simulink model "HCS_function_blocks"  (R2023a)
settings: Solver=ode23t  StartTime=0.0  StopTime=10  RelTol=1e-3
undefined symbols (not defined in the file): Down, Up
libraries: eePwmGenerator x1, spspowerguiLib x1
settings Model: NumberOfSteps=1000  PacingRate=89  Creator=Matt Smith  LastModifiedBy=matty

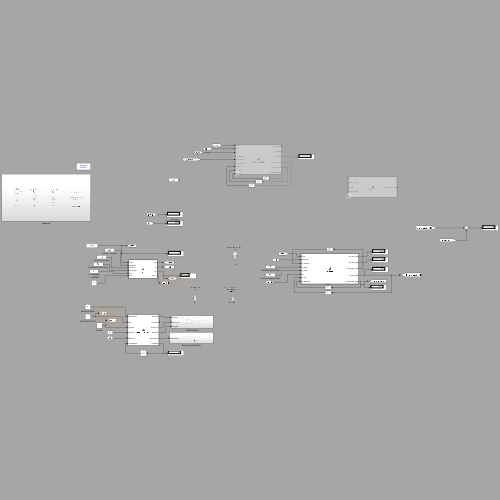
[thumbnail: Simulink's stored preview of the top-level diagram]
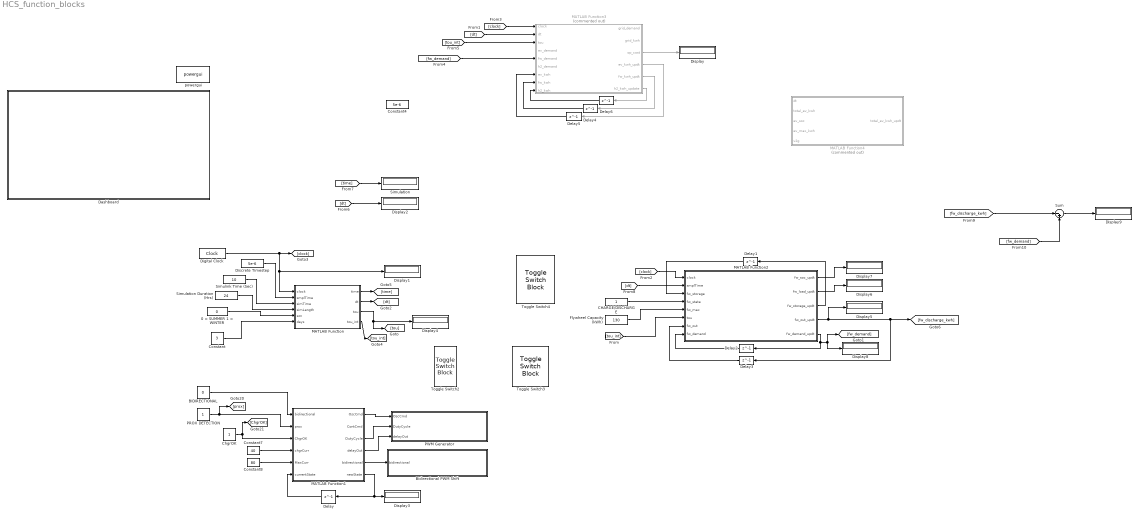
== system HCS_function_blocks ==
  0 = SUMMER 1 = WINTER : Constant  Value=0
  BIDIRECTIONAL : Constant  Value=0
  Bidirectional PWM Shift : Subsystem
  CHARGE/DISCHARGE : Constant
  ChgrOK : Constant
  Constant : Constant  Value=3
  Constant4 : Constant  Value=5e-6
  Constant7 : Constant  Value=40
  Constant8 : Constant  Value=80
  Dashboard : Subsystem
  Delay : Delay  DelayLength=1  InitialCondition=0
  Delay{1..6} (6 alike) : Delay  DelayLength=1  SampleTime=5e-6
  Digital Clock : DigitalClock  SampleTime=5e-6
  Discrete Timestep : Constant  Value=5e-6
  Display{,1..9} (10 alike) : Display
  Flywheel Capacity (kWh) : Constant  Value=130
  MATLAB Function : MATLAB Function  TreatAsAtomicUnit=on
  MATLAB Function1 : MATLAB Function  TreatAsAtomicUnit=on
  MATLAB Function2 : MATLAB Function  TreatAsAtomicUnit=on
  MATLAB Function3 : MATLAB Function  Commented=on  TreatAsAtomicUnit=on
  MATLAB Function4 : MATLAB Function  Commented=on  TreatAsAtomicUnit=on
  PROX DETECTION : Constant
  PWM Generator : Subsystem
  Simulation : Display
  Simulation Duration (Hrs) : Constant  Value=24
  Simulink Time (Sec) : Constant  Value=10
  Sum : Sum  Inputs=|-+
  Toggle Switch2 : ToggleSwitchBlock
      settings: Values={{'Off', 'On'}, [0 1]}
  Toggle Switch3 : ToggleSwitchBlock
      settings: Values={{'SUMMER', 'WINTER'}, [0 1]}
  Toggle Switch4 : ToggleSwitchBlock
      settings: Values={{'Off', 'On'}, [-1 1]}
  powergui : spspowerguiLib/powergui  Priority=1  SimulationMode=Discrete  SampleTime=5e-6  frequency=60  Iterations=50  frequencyindice=0  Pbase=100e6  ErrMax=1e-4  UnitsV=kV  UnitsW=MW  buscounter=0  FunctionMessages=off  echomessages=off  EnableUseOfTLC=off  CurrentSourceSwitches=off  DisableSnubberDevices=off  DisableRonSwitches=off  DisableVfSwitches=off  DisplayEquations=off  AutomaticDiscreteSolvers=off  SolverType=Tustin/Backward Euler (TBE)  Interpol=off  ExternalGateDelay=off  methode=off  Ts=100  x0status=blocks  SPID=on  SwTol=0  HookPort=off  NonlinearTolerance=1e-4  nMaxIteration=100  ContinueOnMaxIteration=off  RestoreLinks=warning  ResistiveCurrentMeasurement=off  Frange=[0:2:500]  Ylog=off  Xlog=on  ShowGrid=off  save=off  variable=ZData  structure=0  ZoomFFT=off  StartTime=0.0  cycles=1  DisplayStyle=1  fundamental=60  FreqAxis=off  MaxFrequency=1000  frequencyindicesteady=1  RmsSteady=1  display=off
  wires:
  Constant8/1 -> MATLAB Function1/5(MaxCurr)
  PROX DETECTION/1 -> MATLAB Function1/2(prox), [prox]
  Constant7/1 -> MATLAB Function1/4(chgrCurr)
  BIDIRECTIONAL/1 -> MATLAB Function1/1("bidirectional ")
  Delay/1 -> MATLAB Function1/6(currentState)
  ChgrOK/1 -> [ChgrOK], MATLAB Function1/3(ChgrOK)
  MATLAB Function1/6(newState) -> Delay/1, Display3/1
  MATLAB Function1/5(bidirectional) -> Bidirectional PWM Shift/1(bidirectional)
  MATLAB Function1/1(OscCmd) -> PWM Generator/1(OscCmd)
  MATLAB Function1/4(delayOut) -> PWM Generator/3(delayOut)
  MATLAB Function1/3(DutyCycle) -> PWM Generator/2(DutyCycle)
  Digital Clock/1 -> [clock], MATLAB Function/1(clock), Display1/1
  Discrete Timestep/1 -> MATLAB Function/2(smplTime)
  MATLAB Function/3(tou) -> [tou], Display4/1
  Simulink Time (Sec)/1 -> MATLAB Function/3(simTime)
  Simulation Duration (Hrs)/1 -> MATLAB Function/4(simLength)
  0 = SUMMER 1 = WINTER/1 -> MATLAB Function/5(szn)
  [tou_int] -> MATLAB Function2/6(tou)
  MATLAB Function2/3(fw_storage_updt) -> Delay1/1
  Delay1/1 -> MATLAB Function2/3(fw_storage)
  Flywheel Capacity (kWh)/1 -> MATLAB Function2/5(fw_max)
  MATLAB Function2/4(fw_out_updt) -> [fw_discharge_kwh], Delay3/1, Display5/1
  MATLAB Function2/2(fw_load_updt) -> Display6/1
  MATLAB Function2/1(fw_soc_updt) -> Display7/1
  MATLAB Function2/5(fw_demand_updt) -> Delay2/1, [fw_demand], Display8/1
  MATLAB Function/2(dt) -> [dt]
  [clock] -> MATLAB Function2/1(clock)
  Delay2/1 -> MATLAB Function2/8(fw_demand)
  Constant/1 -> MATLAB Function/6(days)
  CHARGE/DISCHARGE/1 -> MATLAB Function2/4(fw_state)
  MATLAB Function/4(tou_int) -> [tou_int]
  [dt] -> MATLAB Function3/2(dt)
  [tou_int] -> MATLAB Function3/3(tou)
  [fw_demand] -> MATLAB Function3/5(fw_demand)
  MATLAB Function3/3(op_cost) -> Display/1
  [clock] -> MATLAB Function3/1(clock)
  [dt] -> Display2/1
  MATLAB Function/1(time) -> [time]
  [time] -> Simulation/1
  [dt] -> MATLAB Function2/2(smplTime)
  Delay3/1 -> MATLAB Function2/7(fw_out)
  [fw_discharge_kwh] -> Sum/1
  [fw_demand] -> Sum/2
  Sum/1 -> Display9/1
  MATLAB Function3/4(ev_kwh_updt) -> Delay5/1
  Delay5/1 -> MATLAB Function3/7(ev_kwh)
  MATLAB Function3/5(fw_kwh_updt) -> Delay4/1
  Delay4/1 -> MATLAB Function3/8(fw_kwh)
  MATLAB Function3/6(h2_kwh_update) -> Delay6/1
  Delay6/1 -> MATLAB Function3/9(h2_kwh)

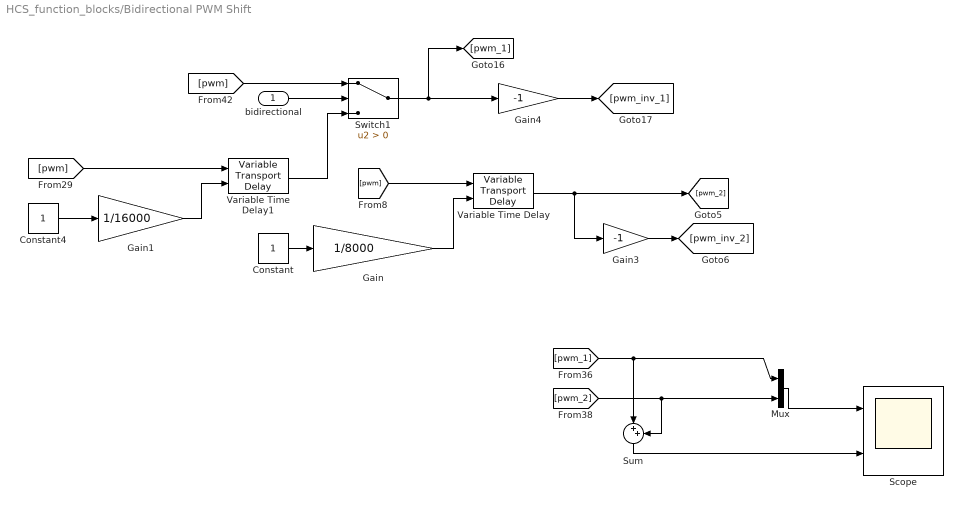
== system HCS_function_blocks/Bidirectional PWM Shift ==
  bidirectional : Inport
  Constant : Constant  SampleTime=5e-6
  Constant4 : Constant  SampleTime=5e-6
  Gain : Gain  Gain=1/8000
  Gain1 : Gain  Gain=1/16000
  Gain3 : Gain  Gain=-1
  Gain4 : Gain  Gain=-1
  Mux : Mux  Inputs=2
  Scope : Scope  NumInputPorts=2
  Sum : Sum  Inputs=|++
  Switch1 : Switch  Criteria=u2 > Threshold  SaturateOnIntegerOverflow=off  InputSameDT=off
  Variable Time Delay : VariableTransportDelay  MaximumDelay=10  MaximumPoints=4096
  Variable Time Delay1 : VariableTransportDelay  MaximumDelay=10  MaximumPoints=12288
  wires:
  Gain/1 -> Variable Time Delay/2
  Variable Time Delay1/1 -> Switch1/3
  Constant4/1 -> Gain1/1
  Gain3/1 -> [pwm_inv_2]
  Gain4/1 -> [pwm_inv_1]
  Variable Time Delay/1 -> Gain3/1, [pwm_2]
  Switch1/1 -> [pwm_1], Gain4/1
  bidirectional/1 -> Switch1/2
  Constant/1 -> Gain/1
  [pwm] -> Variable Time Delay/1
  Gain1/1 -> Variable Time Delay1/2
  [pwm] -> Variable Time Delay1/1
  [pwm] -> Switch1/1
  Mux/1 -> Scope/1
  [pwm_2] -> Mux/2, Sum/2
  [pwm_1] -> Sum/1, Mux/1
  Sum/1 -> Scope/2

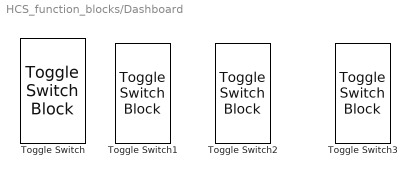
== system HCS_function_blocks/Dashboard ==
  Toggle Switch{,1..3} (4 alike) : ToggleSwitchBlock

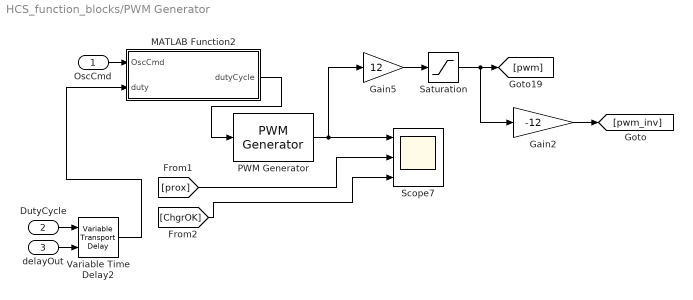
== system HCS_function_blocks/PWM Generator ==
  OscCmd : Inport
  DutyCycle : Inport  Port=2
  delayOut : Inport  Port=3
  Gain2 : Gain  Gain=-12
  Gain5 : Gain  Gain=12
  MATLAB Function2 : MATLAB Function  TreatAsAtomicUnit=on
  PWM Generator : eePwmGenerator/PWM Generator  CarrCount=Up-Down  Tper=1/8000  Tdelay=0  Ts=5e-6
  Saturation : Saturate  UpperLimit=12  LowerLimit=-12  LinearizeAsGain=off
  Scope7 : Scope  NumInputPorts=3
  Variable Time Delay2 : VariableTransportDelay  MaximumDelay=10  MaximumPoints=4096
  wires:
  PWM Generator/1 -> Scope7/1, Gain5/1
  [ChgrOK] -> Scope7/3
  Gain5/1 -> Saturation/1
  Gain2/1 -> [pwm_inv]
  Variable Time Delay2/1 -> MATLAB Function2/2(duty)
  MATLAB Function2/1(dutyCycle) -> PWM Generator/1
  Saturation/1 -> [pwm], Gain2/1
  [prox] -> Scope7/2
  OscCmd/1 -> MATLAB Function2/1(OscCmd)
  delayOut/1 -> Variable Time Delay2/2
  DutyCycle/1 -> Variable Time Delay2/1

== matlab function HCS_function_blocks/MATLAB Function1 ==
  data: OscCmd output; ContCmd output; DutyCycle output; delayOut output; bidirectional output; newState output; bidirectional input; prox input; ChgrOK input; chgrCurr input; MaxCurr input; currentState input
function [OscCmd, ContCmd, DutyCycle, delayOut, bidirectional, newState] = saej1772EVSE(bidirectional, prox, ChgrOK, chgrCurr, MaxCurr, currentState)
% Initialize outputs
        
    OscCmd = 0; ContCmd = 0; DutyCycle = 1; delayOut = 0.001; % Default values for disconnected state
    newState = currentState; % By default, state remains unchanged unless specified

    % Error handling not explicitly defined, so integrating basic checks
    if prox ~= 0 && prox ~= 1 || ChgrOK ~= 0 && ChgrOK ~= 1
        error('Input values for prox and ChgrOK must be either 0 or 1.');
    end
    
    % State A: Disconnected
    if prox == 0
        newState = 1; % STATE A
        
    % State B1: Vehicle connected, not ready to charge, EVSE not ready
    elseif prox == 1 && ChgrOK == 0
        newState = 21; % STATE B1
        
    % Transition between B1 and B2 based on currentState and inputs
    elseif prox == 1 && ChgrOK == 1
        switch int32(currentState)
            case 21
                DutyCycle = 0.05; % EVSE ready, but not charging
                newState = 22; % STATE B2
                delayOut = 0.01;
            case 22
                ContCmd = 1; DutyCycle = 0.05; % Vehicle ready to charge
                newState = 31; % STATE C1
                delayOut = 0.05;
            case 31
                newState = 32; % Connector closed, energy transfer setup, 
                DutyCycle = 0.05; delayOut = 0.1; % STATE C2
            case {32, 33}
                % Actual charging in progress
                newState = 33; % STATE C3
                if chgrCurr >= 6 && chgrCurr <= 51
                    DutyCycle = (chgrCurr/0.6)*0.01;
                elseif chgrCurr > 51 && chgrCurr <= 80
                    DutyCycle = (chgrCurr/2.5 + 64)*0.01;
                end
            otherwise
                % Handle unexpected states or errors by turning off outputs
                ContCmd = 0; DutyCycle = 1; delayOut = 0.001;
                if prox == 1
                    newState = 21; % Return to B1 if error detected but vehicle connected
                                   % STATE B2
                else
                    newState = 1; % Otherwise, return to disconnected state
                                  % STATE A
                end
        end
    end
    
    % Set OscCmd and ContCmd based on newState to reflect final decisions
    %newState = int32(newState);
    switch int32(newState)
        case {22, 31, 32, 33}
            OscCmd = 1; % Oscillator needs to be on for these states
        otherwise
            OscCmd = 0;
    end
    
    % ContCmd is already set in specific state transitions
    % DutyCycle adjustments are made within state transitions
end

== matlab function HCS_function_blocks/MATLAB Function ==
  data: clock input; time output; smplTime input; dt output; tou output; simTime input; simLength input; szn input; days input; tou_int output
function [time, dt, tou, tou_int] = fcn(clock, smplTime, simTime, simLength, szn, days)
    % Adjusted simulation time to span over 'days' days
    % First, calculate the total simulation time in hours for the given number of days
    totalSimHours = simLength * days;
    
    % Convert clock (in seconds) to actual simulation time (in hours)
    % Instead of scaling the entire simulation to fit within a single day,
    % scale it based on the total simulation hours specified by 'days'
    scalingFactor = totalSimHours / (simTime / 3600);
    scaledTime = clock / 3600 * scalingFactor; % Convert clock to hours and scale based on totalSimHours
    
    tou = "null";
    tou_int = 0;

    % Outputs
    time = scaledTime; % The scaled simulation time in hours, adjusted for multiple days
    dt = (smplTime / simTime); % The timestep in hours

    % Determine the time of use (TOU) state based on the scaled simulation time
    % For TOU calculations, use mod(time, 24) to determine the time of day for TOU state decisions
    currentTimeOfDay = mod(time, 24);

    % Assuming the 'hrs' variable represents an hour in the context of currentTimeOfDay
    hrs = 1; % 1 hour in terms of scaled simulation time

    % Update TOU state checks to use currentTimeOfDay for daily cycle logic
    if szn == 0
        if (currentTimeOfDay >= 0*hrs && currentTimeOfDay <= 7*hrs) || (currentTimeOfDay > 19*hrs && currentTimeOfDay <= 24*hrs)
            tou = "off_peak";
            tou_int = 1; % off peak
        elseif (currentTimeOfDay > 7*hrs && currentTimeOfDay <= 11*hrs)
            tou = "mid_peak_hi";
            tou_int = 3; % mid peak hi
        elseif (currentTimeOfDay > 11*hrs && currentTimeOfDay <= 17*hrs)
            tou = "on_peak";
            tou_int = 4; % on peak
        elseif (currentTimeOfDay > 17*hrs && currentTimeOfDay <= 19*hrs)
            tou = "mid_peak_lo";
            tou_int = 2; % mid peak lo
        else
            tou = "null";
            tou_int = 0; % null/error
        end
    elseif szn == 1
        if (currentTimeOfDay >= 0*hrs && currentTimeOfDay <= 7*hrs) || (currentTimeOfDay > 19*hrs && currentTimeOfDay <= 24*hrs)
            tou = "off_peak";
            tou_int = 1; % off peak
        elseif (currentTimeOfDay > 7*hrs && currentTimeOfDay <= 11*hrs)
            tou = "on_peak";
            tou_int = 4; % on peak
        elseif (currentTimeOfDay > 11*hrs && currentTimeOfDay <= 17*hrs)
            tou = "mid_peak_lo";
            tou_int = 2; % mid peak lo
        elseif (currentTimeOfDay > 17*hrs && currentTimeOfDay <= 19*hrs)
            tou = "on_peak";
            tou_int = 4; % on peak
        else
            tou = "null";
        end
    end 
end

== matlab function HCS_function_blocks/PWM Generator/MATLAB Function2 ==
  data: OscCmd input; dutyCycle output; duty input
function dutyCycle = oscCheck(OscCmd, duty)
if OscCmd == 1
    dutyCycle = duty;
else
    dutyCycle = 1;
end

== matlab function HCS_function_blocks/MATLAB Function2 ==
  data: clock input; smplTime input; fw_soc_updt output; fw_storage input; fw_state input; fw_max input; tou input; fw_out input; fw_load_updt output; fw_storage_updt output; fw_out_updt output; fw_demand_updt output; fw_demand input
function [fw_soc_updt, fw_load_updt, fw_storage_updt, fw_out_updt, fw_demand_updt] = flywheel(clock, smplTime, fw_storage, fw_state, fw_max, tou, fw_out, fw_demand)
    % Initialize output
    
    % Calculate current state of charge (SoC)
    fw_soc = fw_storage / fw_max * 100; % in percentage

    switch tou
        case 4
            if fw_state > 0 % Manual kill switch
                fw_load_updt = -abs(250*fw_state); % Discharge (negative load)
            else
                fw_load_updt = 0; % Do not discharge
            end
        case {2, 3}
            if fw_state > 0 && fw_storage < fw_max
                fw_load_updt = abs(250*fw_state); % Charge (positive load)
            else
                fw_load_updt = 0; % Do not charge if at max capacity
            end
        case 1
            % Charging conditions
            if fw_state > 0 && fw_storage < fw_max
                fw_load_updt = abs(250*fw_state); % Charge (positive load)
            else
                fw_load_updt = 0; % Do not charge if at max capacity
            end
        otherwise
            if fw_state > 0 && fw_storage < fw_max
                fw_load_updt = abs(250*fw_state); % Charge (positive load)
            else
                fw_load_updt = 0; % Do not charge if at max capacity
            end
    end
    
    % Uncomment the following lines for station demand logic when threshold is defined
    % if station_demand > <defined_threshold>
    %     fw_load_updt = -abs(fw_state); % Discharge to meet high station demand
    % end
    
    % Update flywheel storage and SoC based on load update
    fw_storage_updt = fw_storage + (fw_load_updt * smplTime); % Convert kW to kWh using smplTime, assuming smplTime is in hours
    fw_soc_updt = fw_storage_updt / fw_max * 100; % Update SoC
    
    % Accumulate energy supplied to station by the flywheel
    if fw_load_updt < 0 % If discharging
        fw_out_updt = fw_out - fw_load_updt * smplTime; % Convert kW to kWh, accumulate discharge only
        fw_demand_updt = fw_demand;
    elseif fw_load_updt > 0
        fw_out_updt = fw_out;
        fw_demand_updt = fw_demand + (fw_load_updt * smplTime);
    else
        fw_out_updt = fw_out;
        fw_demand_updt = fw_demand;
    end

end

== matlab function HCS_function_blocks/MATLAB Function3 ==
  data: clock input; grid_demand output; grid_kwh output; dt input; tou input; ev_demand input; fw_demand input; h2_demand input; op_cost output; ev_kwh input; fw_kwh input; ev_kwh_updt output; fw_kwh_updt output; h2_kwh input; h2_kwh_update output
function [grid_demand, grid_kwh, op_cost, ev_kwh_updt, fw_kwh_updt, h2_kwh_update] = station_monitor(clock, dt, tou, ev_demand, fw_demand, h2_demand, ev_kwh, fw_kwh, h2_kwh)
% INPUTS:
% clock = Either Simulink simulation time (in seconds) or the scaled simulation time (in hours)
% dt = Scaled simulation step size (in hours)
% tou = time of use
% 	{	0 - null/error value
% 		1 - off_peak
% 		2 - mid_peak_lo
% 		3 - mid_peak_hi
% 		4 - on_peak	}
% ev_demand = Electricity supplied from the power grid to connected EV(s) (in kW)
% fw_demand = Electricity supplied by or discharged to the power grid, depending on flywheel SOC and state
% ev_kwh = Running total of kWh consumed by connected EV(s)
% fw_kwh = Running tota of kWh consumed by or discharged from flywheel
% 
% OUTPUTS:
% grid_demand = the sum of immediate grid demand (i.e., the sum of kW supplied by the grid to other system components
% grid_kwh = The running total of kWh consumed by the station
% op_cost = Operational cost of station (running total, calculate using grid_kwh)
% 	{	tou = 0: cost is 0 cents an hour (tou = 0 is a null value)
% 		tou = 1: cost is 0.087 cents per kWh
% 		tou = 2: cost is 0.122 cents per kWh
% 		tou = 3: cost is 0.122 cents per kWh
% 		tou = 4: cost is 0.182 cents per kWh }
% ev_kwh_updt = Updated running total of kWh consumed by (or supplied back to grid, via V2G) EVs
% fw_kwh_updt = Update running total of kWh consumed (or supplied to grid) by flywheel

    % Calculate immediate grid demand
    grid_demand = ev_demand + fw_demand;

    % Update running totals for kWh
    ev_kwh_updt = ev_kwh + (ev_demand * dt);
    fw_kwh_updt = fw_kwh + (fw_demand * dt);
    h2_kwh_update = h2_kwh + (h2_demand * dt);

    % Update the station's total kWh consumption
    grid_kwh = ev_kwh_updt + fw_kwh_updt;

    % Determine operational cost based on TOU
    switch tou
        case 1
            cost_per_kWh = 0.087;
        case {2, 3}
            cost_per_kWh = 0.122;
        case 4
            cost_per_kWh = 0.182;
        otherwise
            cost_per_kWh = 0;
    end

    % Calculate operational cost
    op_cost = grid_kwh * cost_per_kWh;

end

== matlab function HCS_function_blocks/MATLAB Function4 ==
  data: dt input; total_ev_kwh_updt output; total_ev_kwh input; ev_soc input; ev_max_kwh input; v2g input
function total_ev_kwh_updt  = ev_monitor(dt, total_ev_kwh, ev_soc, ev_max_kwh, v2g)

end
